simulink model "test2"  (R2020b)
settings: Solver=FixedStepAuto  StartTime=0.0  StopTime=10.0  RelTol=1e-3
model workspace (MAT data in the model file):
  HDLVAXIMasterConfig : hdlverifier.internal.AXIMaster.ConfigParams (value not decoded)
libraries: hdlsllib x38
(part 2 of 2)

== system test2/AesEnc/ram44by32bit/Subsystem ==
  we : Inport  OutDataTypeStr=boolean
  data1 : Inport  Port=2  OutDataTypeStr=uint32
  data2 : Inport  Port=3  OutDataTypeStr=uint32
  Constant : Constant
  Constant1 : Constant  Value=2
  Dual Rate Dual Port RAM : hdlsllib/HDL RAMs/Dual Rate Dual Port RAM  ram_size=2
      settings: SourceProductBaseCode=SL
  temp_state : Outport  OutDataTypeStr=uint32  VectorParamsAs1DForOutWhenUnconnected=off
  temp_state1 : Outport  Port=2  OutDataTypeStr=uint32  VectorParamsAs1DForOutWhenUnconnected=off
  wires:
  Dual Rate Dual Port RAM/1 -> temp_state/1
  data2/1 -> Dual Rate Dual Port RAM/4
  Constant/1 -> Dual Rate Dual Port RAM/2
  data1/1 -> Dual Rate Dual Port RAM/1
  we/1 -> Dual Rate Dual Port RAM/6, Dual Rate Dual Port RAM/3
  Dual Rate Dual Port RAM/2 -> temp_state1/1
  Constant1/1 -> Dual Rate Dual Port RAM/5

== system test2/AesEnc/ram44by32bit/Subsystem1 ==
  we : Inport  OutDataTypeStr=boolean
  data1 : Inport  Port=2  OutDataTypeStr=uint32
  data2 : Inport  Port=3  OutDataTypeStr=uint32
  Constant : Constant
  Constant1 : Constant  Value=2
  Dual Rate Dual Port RAM : hdlsllib/HDL RAMs/Dual Rate Dual Port RAM  ram_size=2
      settings: SourceProductBaseCode=SL
  temp_state : Outport  OutDataTypeStr=uint32  VectorParamsAs1DForOutWhenUnconnected=off
  temp_state1 : Outport  Port=2  OutDataTypeStr=uint32  VectorParamsAs1DForOutWhenUnconnected=off
  wires:
  Dual Rate Dual Port RAM/1 -> temp_state/1
  data2/1 -> Dual Rate Dual Port RAM/4
  Constant/1 -> Dual Rate Dual Port RAM/2
  data1/1 -> Dual Rate Dual Port RAM/1
  we/1 -> Dual Rate Dual Port RAM/6, Dual Rate Dual Port RAM/3
  Dual Rate Dual Port RAM/2 -> temp_state1/1
  Constant1/1 -> Dual Rate Dual Port RAM/5

== system test2/AesEnc/ram44by32bit/Subsystem10 ==
  we : Inport  OutDataTypeStr=boolean
  data1 : Inport  Port=2  OutDataTypeStr=uint32
  data2 : Inport  Port=3  OutDataTypeStr=uint32
  Constant : Constant
  Constant1 : Constant  Value=2
  Dual Rate Dual Port RAM : hdlsllib/HDL RAMs/Dual Rate Dual Port RAM  ram_size=2
      settings: SourceProductBaseCode=SL
  temp_state : Outport  OutDataTypeStr=uint32  VectorParamsAs1DForOutWhenUnconnected=off
  temp_state1 : Outport  Port=2  OutDataTypeStr=uint32  VectorParamsAs1DForOutWhenUnconnected=off
  wires:
  Dual Rate Dual Port RAM/1 -> temp_state/1
  data2/1 -> Dual Rate Dual Port RAM/4
  Constant/1 -> Dual Rate Dual Port RAM/2
  data1/1 -> Dual Rate Dual Port RAM/1
  we/1 -> Dual Rate Dual Port RAM/6, Dual Rate Dual Port RAM/3
  Dual Rate Dual Port RAM/2 -> temp_state1/1
  Constant1/1 -> Dual Rate Dual Port RAM/5

== system test2/AesEnc/ram44by32bit/Subsystem11 ==
  we : Inport  OutDataTypeStr=boolean
  data1 : Inport  Port=2  OutDataTypeStr=uint32
  data2 : Inport  Port=3  OutDataTypeStr=uint32
  Constant : Constant
  Constant1 : Constant  Value=2
  Dual Rate Dual Port RAM : hdlsllib/HDL RAMs/Dual Rate Dual Port RAM  ram_size=2
      settings: SourceProductBaseCode=SL
  temp_state : Outport  OutDataTypeStr=uint32  VectorParamsAs1DForOutWhenUnconnected=off
  temp_state1 : Outport  Port=2  OutDataTypeStr=uint32  VectorParamsAs1DForOutWhenUnconnected=off
  wires:
  Dual Rate Dual Port RAM/1 -> temp_state/1
  data2/1 -> Dual Rate Dual Port RAM/4
  Constant/1 -> Dual Rate Dual Port RAM/2
  data1/1 -> Dual Rate Dual Port RAM/1
  we/1 -> Dual Rate Dual Port RAM/6, Dual Rate Dual Port RAM/3
  Dual Rate Dual Port RAM/2 -> temp_state1/1
  Constant1/1 -> Dual Rate Dual Port RAM/5

== system test2/AesEnc/ram44by32bit/Subsystem12 ==
  we : Inport  OutDataTypeStr=boolean
  data1 : Inport  Port=2  OutDataTypeStr=uint32
  data2 : Inport  Port=3  OutDataTypeStr=uint32
  Constant : Constant
  Constant1 : Constant  Value=2
  Dual Rate Dual Port RAM : hdlsllib/HDL RAMs/Dual Rate Dual Port RAM  ram_size=2
      settings: SourceProductBaseCode=SL
  temp_state : Outport  OutDataTypeStr=uint32  VectorParamsAs1DForOutWhenUnconnected=off
  temp_state1 : Outport  Port=2  OutDataTypeStr=uint32  VectorParamsAs1DForOutWhenUnconnected=off
  wires:
  Dual Rate Dual Port RAM/1 -> temp_state/1
  data2/1 -> Dual Rate Dual Port RAM/4
  Constant/1 -> Dual Rate Dual Port RAM/2
  data1/1 -> Dual Rate Dual Port RAM/1
  we/1 -> Dual Rate Dual Port RAM/6, Dual Rate Dual Port RAM/3
  Dual Rate Dual Port RAM/2 -> temp_state1/1
  Constant1/1 -> Dual Rate Dual Port RAM/5

== system test2/AesEnc/ram44by32bit/Subsystem13 ==
  we : Inport  OutDataTypeStr=boolean
  data1 : Inport  Port=2  OutDataTypeStr=uint32
  data2 : Inport  Port=3  OutDataTypeStr=uint32
  Constant : Constant
  Constant1 : Constant  Value=2
  Dual Rate Dual Port RAM : hdlsllib/HDL RAMs/Dual Rate Dual Port RAM  ram_size=2
      settings: SourceProductBaseCode=SL
  temp_state : Outport  OutDataTypeStr=uint32  VectorParamsAs1DForOutWhenUnconnected=off
  temp_state1 : Outport  Port=2  OutDataTypeStr=uint32  VectorParamsAs1DForOutWhenUnconnected=off
  wires:
  Dual Rate Dual Port RAM/1 -> temp_state/1
  data2/1 -> Dual Rate Dual Port RAM/4
  Constant/1 -> Dual Rate Dual Port RAM/2
  data1/1 -> Dual Rate Dual Port RAM/1
  we/1 -> Dual Rate Dual Port RAM/6, Dual Rate Dual Port RAM/3
  Dual Rate Dual Port RAM/2 -> temp_state1/1
  Constant1/1 -> Dual Rate Dual Port RAM/5

== system test2/AesEnc/ram44by32bit/Subsystem14 ==
  we : Inport  OutDataTypeStr=boolean
  data1 : Inport  Port=2  OutDataTypeStr=uint32
  data2 : Inport  Port=3  OutDataTypeStr=uint32
  Constant : Constant
  Constant1 : Constant  Value=2
  Dual Rate Dual Port RAM : hdlsllib/HDL RAMs/Dual Rate Dual Port RAM  ram_size=2
      settings: SourceProductBaseCode=SL
  temp_state : Outport  OutDataTypeStr=uint32  VectorParamsAs1DForOutWhenUnconnected=off
  temp_state1 : Outport  Port=2  OutDataTypeStr=uint32  VectorParamsAs1DForOutWhenUnconnected=off
  wires:
  Dual Rate Dual Port RAM/1 -> temp_state/1
  data2/1 -> Dual Rate Dual Port RAM/4
  Constant/1 -> Dual Rate Dual Port RAM/2
  data1/1 -> Dual Rate Dual Port RAM/1
  we/1 -> Dual Rate Dual Port RAM/6, Dual Rate Dual Port RAM/3
  Dual Rate Dual Port RAM/2 -> temp_state1/1
  Constant1/1 -> Dual Rate Dual Port RAM/5

== system test2/AesEnc/ram44by32bit/Subsystem15 ==
  we : Inport  OutDataTypeStr=boolean
  data1 : Inport  Port=2  OutDataTypeStr=uint32
  data2 : Inport  Port=3  OutDataTypeStr=uint32
  Constant : Constant
  Constant1 : Constant  Value=2
  Dual Rate Dual Port RAM : hdlsllib/HDL RAMs/Dual Rate Dual Port RAM  ram_size=2
      settings: SourceProductBaseCode=SL
  temp_state : Outport  OutDataTypeStr=uint32  VectorParamsAs1DForOutWhenUnconnected=off
  temp_state1 : Outport  Port=2  OutDataTypeStr=uint32  VectorParamsAs1DForOutWhenUnconnected=off
  wires:
  Dual Rate Dual Port RAM/1 -> temp_state/1
  data2/1 -> Dual Rate Dual Port RAM/4
  Constant/1 -> Dual Rate Dual Port RAM/2
  data1/1 -> Dual Rate Dual Port RAM/1
  we/1 -> Dual Rate Dual Port RAM/6, Dual Rate Dual Port RAM/3
  Dual Rate Dual Port RAM/2 -> temp_state1/1
  Constant1/1 -> Dual Rate Dual Port RAM/5

== system test2/AesEnc/ram44by32bit/Subsystem16 ==
  we : Inport  OutDataTypeStr=boolean
  data1 : Inport  Port=2  OutDataTypeStr=uint32
  data2 : Inport  Port=3  OutDataTypeStr=uint32
  Constant : Constant
  Constant1 : Constant  Value=2
  Dual Rate Dual Port RAM : hdlsllib/HDL RAMs/Dual Rate Dual Port RAM  ram_size=2
      settings: SourceProductBaseCode=SL
  temp_state : Outport  OutDataTypeStr=uint32  VectorParamsAs1DForOutWhenUnconnected=off
  temp_state1 : Outport  Port=2  OutDataTypeStr=uint32  VectorParamsAs1DForOutWhenUnconnected=off
  wires:
  Dual Rate Dual Port RAM/1 -> temp_state/1
  data2/1 -> Dual Rate Dual Port RAM/4
  Constant/1 -> Dual Rate Dual Port RAM/2
  data1/1 -> Dual Rate Dual Port RAM/1
  we/1 -> Dual Rate Dual Port RAM/6, Dual Rate Dual Port RAM/3
  Dual Rate Dual Port RAM/2 -> temp_state1/1
  Constant1/1 -> Dual Rate Dual Port RAM/5

== system test2/AesEnc/ram44by32bit/Subsystem17 ==
  we : Inport  OutDataTypeStr=boolean
  data1 : Inport  Port=2  OutDataTypeStr=uint32
  data2 : Inport  Port=3  OutDataTypeStr=uint32
  Constant : Constant
  Constant1 : Constant  Value=2
  Dual Rate Dual Port RAM : hdlsllib/HDL RAMs/Dual Rate Dual Port RAM  ram_size=2
      settings: SourceProductBaseCode=SL
  temp_state : Outport  OutDataTypeStr=uint32  VectorParamsAs1DForOutWhenUnconnected=off
  temp_state1 : Outport  Port=2  OutDataTypeStr=uint32  VectorParamsAs1DForOutWhenUnconnected=off
  wires:
  Dual Rate Dual Port RAM/1 -> temp_state/1
  data2/1 -> Dual Rate Dual Port RAM/4
  Constant/1 -> Dual Rate Dual Port RAM/2
  data1/1 -> Dual Rate Dual Port RAM/1
  we/1 -> Dual Rate Dual Port RAM/6, Dual Rate Dual Port RAM/3
  Dual Rate Dual Port RAM/2 -> temp_state1/1
  Constant1/1 -> Dual Rate Dual Port RAM/5

== system test2/AesEnc/ram44by32bit/Subsystem18 ==
  we : Inport  OutDataTypeStr=boolean
  data1 : Inport  Port=2  OutDataTypeStr=uint32
  data2 : Inport  Port=3  OutDataTypeStr=uint32
  Constant : Constant
  Constant1 : Constant  Value=2
  Dual Rate Dual Port RAM : hdlsllib/HDL RAMs/Dual Rate Dual Port RAM  ram_size=2
      settings: SourceProductBaseCode=SL
  temp_state : Outport  OutDataTypeStr=uint32  VectorParamsAs1DForOutWhenUnconnected=off
  temp_state1 : Outport  Port=2  OutDataTypeStr=uint32  VectorParamsAs1DForOutWhenUnconnected=off
  wires:
  Dual Rate Dual Port RAM/1 -> temp_state/1
  data2/1 -> Dual Rate Dual Port RAM/4
  Constant/1 -> Dual Rate Dual Port RAM/2
  data1/1 -> Dual Rate Dual Port RAM/1
  we/1 -> Dual Rate Dual Port RAM/6, Dual Rate Dual Port RAM/3
  Dual Rate Dual Port RAM/2 -> temp_state1/1
  Constant1/1 -> Dual Rate Dual Port RAM/5

== system test2/AesEnc/ram44by32bit/Subsystem19 ==
  we : Inport  OutDataTypeStr=boolean
  data1 : Inport  Port=2  OutDataTypeStr=uint32
  data2 : Inport  Port=3  OutDataTypeStr=uint32
  Constant : Constant
  Constant1 : Constant  Value=2
  Dual Rate Dual Port RAM : hdlsllib/HDL RAMs/Dual Rate Dual Port RAM  ram_size=2
      settings: SourceProductBaseCode=SL
  temp_state : Outport  OutDataTypeStr=uint32  VectorParamsAs1DForOutWhenUnconnected=off
  temp_state1 : Outport  Port=2  OutDataTypeStr=uint32  VectorParamsAs1DForOutWhenUnconnected=off
  wires:
  Dual Rate Dual Port RAM/1 -> temp_state/1
  data2/1 -> Dual Rate Dual Port RAM/4
  Constant/1 -> Dual Rate Dual Port RAM/2
  data1/1 -> Dual Rate Dual Port RAM/1
  we/1 -> Dual Rate Dual Port RAM/6, Dual Rate Dual Port RAM/3
  Dual Rate Dual Port RAM/2 -> temp_state1/1
  Constant1/1 -> Dual Rate Dual Port RAM/5

== system test2/AesEnc/ram44by32bit/Subsystem2 ==
  we : Inport  OutDataTypeStr=boolean
  data1 : Inport  Port=2  OutDataTypeStr=uint32
  data2 : Inport  Port=3  OutDataTypeStr=uint32
  Constant : Constant
  Constant1 : Constant  Value=2
  Dual Rate Dual Port RAM : hdlsllib/HDL RAMs/Dual Rate Dual Port RAM  ram_size=2
      settings: SourceProductBaseCode=SL
  temp_state : Outport  OutDataTypeStr=uint32  VectorParamsAs1DForOutWhenUnconnected=off
  temp_state1 : Outport  Port=2  OutDataTypeStr=uint32  VectorParamsAs1DForOutWhenUnconnected=off
  wires:
  Dual Rate Dual Port RAM/1 -> temp_state/1
  data2/1 -> Dual Rate Dual Port RAM/4
  Constant/1 -> Dual Rate Dual Port RAM/2
  data1/1 -> Dual Rate Dual Port RAM/1
  we/1 -> Dual Rate Dual Port RAM/6, Dual Rate Dual Port RAM/3
  Dual Rate Dual Port RAM/2 -> temp_state1/1
  Constant1/1 -> Dual Rate Dual Port RAM/5

== system test2/AesEnc/ram44by32bit/Subsystem20 ==
  we : Inport  OutDataTypeStr=boolean
  data1 : Inport  Port=2  OutDataTypeStr=uint32
  data2 : Inport  Port=3  OutDataTypeStr=uint32
  Constant : Constant
  Constant1 : Constant  Value=2
  Dual Rate Dual Port RAM : hdlsllib/HDL RAMs/Dual Rate Dual Port RAM  ram_size=2
      settings: SourceProductBaseCode=SL
  temp_state : Outport  OutDataTypeStr=uint32  VectorParamsAs1DForOutWhenUnconnected=off
  temp_state1 : Outport  Port=2  OutDataTypeStr=uint32  VectorParamsAs1DForOutWhenUnconnected=off
  wires:
  Dual Rate Dual Port RAM/1 -> temp_state/1
  data2/1 -> Dual Rate Dual Port RAM/4
  Constant/1 -> Dual Rate Dual Port RAM/2
  data1/1 -> Dual Rate Dual Port RAM/1
  we/1 -> Dual Rate Dual Port RAM/6, Dual Rate Dual Port RAM/3
  Dual Rate Dual Port RAM/2 -> temp_state1/1
  Constant1/1 -> Dual Rate Dual Port RAM/5

== system test2/AesEnc/ram44by32bit/Subsystem21 ==
  we : Inport  OutDataTypeStr=boolean
  data1 : Inport  Port=2  OutDataTypeStr=uint32
  data2 : Inport  Port=3  OutDataTypeStr=uint32
  Constant : Constant
  Constant1 : Constant  Value=2
  Dual Rate Dual Port RAM : hdlsllib/HDL RAMs/Dual Rate Dual Port RAM  ram_size=2
      settings: SourceProductBaseCode=SL
  temp_state : Outport  OutDataTypeStr=uint32  VectorParamsAs1DForOutWhenUnconnected=off
  temp_state1 : Outport  Port=2  OutDataTypeStr=uint32  VectorParamsAs1DForOutWhenUnconnected=off
  wires:
  Dual Rate Dual Port RAM/1 -> temp_state/1
  data2/1 -> Dual Rate Dual Port RAM/4
  Constant/1 -> Dual Rate Dual Port RAM/2
  data1/1 -> Dual Rate Dual Port RAM/1
  we/1 -> Dual Rate Dual Port RAM/6, Dual Rate Dual Port RAM/3
  Dual Rate Dual Port RAM/2 -> temp_state1/1
  Constant1/1 -> Dual Rate Dual Port RAM/5

== system test2/AesEnc/ram44by32bit/Subsystem3 ==
  we : Inport  OutDataTypeStr=boolean
  data1 : Inport  Port=2  OutDataTypeStr=uint32
  data2 : Inport  Port=3  OutDataTypeStr=uint32
  Constant : Constant
  Constant1 : Constant  Value=2
  Dual Rate Dual Port RAM : hdlsllib/HDL RAMs/Dual Rate Dual Port RAM  ram_size=2
      settings: SourceProductBaseCode=SL
  temp_state : Outport  OutDataTypeStr=uint32  VectorParamsAs1DForOutWhenUnconnected=off
  temp_state1 : Outport  Port=2  OutDataTypeStr=uint32  VectorParamsAs1DForOutWhenUnconnected=off
  wires:
  Dual Rate Dual Port RAM/1 -> temp_state/1
  data2/1 -> Dual Rate Dual Port RAM/4
  Constant/1 -> Dual Rate Dual Port RAM/2
  data1/1 -> Dual Rate Dual Port RAM/1
  we/1 -> Dual Rate Dual Port RAM/6, Dual Rate Dual Port RAM/3
  Dual Rate Dual Port RAM/2 -> temp_state1/1
  Constant1/1 -> Dual Rate Dual Port RAM/5

== system test2/AesEnc/ram44by32bit/Subsystem4 ==
  we : Inport  OutDataTypeStr=boolean
  data1 : Inport  Port=2  OutDataTypeStr=uint32
  data2 : Inport  Port=3  OutDataTypeStr=uint32
  Constant : Constant
  Constant1 : Constant  Value=2
  Dual Rate Dual Port RAM : hdlsllib/HDL RAMs/Dual Rate Dual Port RAM  ram_size=2
      settings: SourceProductBaseCode=SL
  temp_state : Outport  OutDataTypeStr=uint32  VectorParamsAs1DForOutWhenUnconnected=off
  temp_state1 : Outport  Port=2  OutDataTypeStr=uint32  VectorParamsAs1DForOutWhenUnconnected=off
  wires:
  Dual Rate Dual Port RAM/1 -> temp_state/1
  data2/1 -> Dual Rate Dual Port RAM/4
  Constant/1 -> Dual Rate Dual Port RAM/2
  data1/1 -> Dual Rate Dual Port RAM/1
  we/1 -> Dual Rate Dual Port RAM/6, Dual Rate Dual Port RAM/3
  Dual Rate Dual Port RAM/2 -> temp_state1/1
  Constant1/1 -> Dual Rate Dual Port RAM/5

== system test2/AesEnc/ram44by32bit/Subsystem5 ==
  we : Inport  OutDataTypeStr=boolean
  data1 : Inport  Port=2  OutDataTypeStr=uint32
  data2 : Inport  Port=3  OutDataTypeStr=uint32
  Constant : Constant
  Constant1 : Constant  Value=2
  Dual Rate Dual Port RAM : hdlsllib/HDL RAMs/Dual Rate Dual Port RAM  ram_size=2
      settings: SourceProductBaseCode=SL
  temp_state : Outport  OutDataTypeStr=uint32  VectorParamsAs1DForOutWhenUnconnected=off
  temp_state1 : Outport  Port=2  OutDataTypeStr=uint32  VectorParamsAs1DForOutWhenUnconnected=off
  wires:
  Dual Rate Dual Port RAM/1 -> temp_state/1
  data2/1 -> Dual Rate Dual Port RAM/4
  Constant/1 -> Dual Rate Dual Port RAM/2
  data1/1 -> Dual Rate Dual Port RAM/1
  we/1 -> Dual Rate Dual Port RAM/6, Dual Rate Dual Port RAM/3
  Dual Rate Dual Port RAM/2 -> temp_state1/1
  Constant1/1 -> Dual Rate Dual Port RAM/5

== system test2/AesEnc/ram44by32bit/Subsystem6 ==
  we : Inport  OutDataTypeStr=boolean
  data1 : Inport  Port=2  OutDataTypeStr=uint32
  data2 : Inport  Port=3  OutDataTypeStr=uint32
  Constant : Constant
  Constant1 : Constant  Value=2
  Dual Rate Dual Port RAM : hdlsllib/HDL RAMs/Dual Rate Dual Port RAM  ram_size=2
      settings: SourceProductBaseCode=SL
  temp_state : Outport  OutDataTypeStr=uint32  VectorParamsAs1DForOutWhenUnconnected=off
  temp_state1 : Outport  Port=2  OutDataTypeStr=uint32  VectorParamsAs1DForOutWhenUnconnected=off
  wires:
  Dual Rate Dual Port RAM/1 -> temp_state/1
  data2/1 -> Dual Rate Dual Port RAM/4
  Constant/1 -> Dual Rate Dual Port RAM/2
  data1/1 -> Dual Rate Dual Port RAM/1
  we/1 -> Dual Rate Dual Port RAM/6, Dual Rate Dual Port RAM/3
  Dual Rate Dual Port RAM/2 -> temp_state1/1
  Constant1/1 -> Dual Rate Dual Port RAM/5

== system test2/AesEnc/ram44by32bit/Subsystem7 ==
  we : Inport  OutDataTypeStr=boolean
  data1 : Inport  Port=2  OutDataTypeStr=uint32
  data2 : Inport  Port=3  OutDataTypeStr=uint32
  Constant : Constant
  Constant1 : Constant  Value=2
  Dual Rate Dual Port RAM : hdlsllib/HDL RAMs/Dual Rate Dual Port RAM  ram_size=2
      settings: SourceProductBaseCode=SL
  temp_state : Outport  OutDataTypeStr=uint32  VectorParamsAs1DForOutWhenUnconnected=off
  temp_state1 : Outport  Port=2  OutDataTypeStr=uint32  VectorParamsAs1DForOutWhenUnconnected=off
  wires:
  Dual Rate Dual Port RAM/1 -> temp_state/1
  data2/1 -> Dual Rate Dual Port RAM/4
  Constant/1 -> Dual Rate Dual Port RAM/2
  data1/1 -> Dual Rate Dual Port RAM/1
  we/1 -> Dual Rate Dual Port RAM/6, Dual Rate Dual Port RAM/3
  Dual Rate Dual Port RAM/2 -> temp_state1/1
  Constant1/1 -> Dual Rate Dual Port RAM/5

== system test2/AesEnc/ram44by32bit/Subsystem8 ==
  we : Inport  OutDataTypeStr=boolean
  data1 : Inport  Port=2  OutDataTypeStr=uint32
  data2 : Inport  Port=3  OutDataTypeStr=uint32
  Constant : Constant
  Constant1 : Constant  Value=2
  Dual Rate Dual Port RAM : hdlsllib/HDL RAMs/Dual Rate Dual Port RAM  ram_size=2
      settings: SourceProductBaseCode=SL
  temp_state : Outport  OutDataTypeStr=uint32  VectorParamsAs1DForOutWhenUnconnected=off
  temp_state1 : Outport  Port=2  OutDataTypeStr=uint32  VectorParamsAs1DForOutWhenUnconnected=off
  wires:
  Dual Rate Dual Port RAM/1 -> temp_state/1
  data2/1 -> Dual Rate Dual Port RAM/4
  Constant/1 -> Dual Rate Dual Port RAM/2
  data1/1 -> Dual Rate Dual Port RAM/1
  we/1 -> Dual Rate Dual Port RAM/6, Dual Rate Dual Port RAM/3
  Dual Rate Dual Port RAM/2 -> temp_state1/1
  Constant1/1 -> Dual Rate Dual Port RAM/5

== system test2/AesEnc/ram44by32bit/Subsystem9 ==
  we : Inport  OutDataTypeStr=boolean
  data1 : Inport  Port=2  OutDataTypeStr=uint32
  data2 : Inport  Port=3  OutDataTypeStr=uint32
  Constant : Constant
  Constant1 : Constant  Value=2
  Dual Rate Dual Port RAM : hdlsllib/HDL RAMs/Dual Rate Dual Port RAM  ram_size=2
      settings: SourceProductBaseCode=SL
  temp_state : Outport  OutDataTypeStr=uint32  VectorParamsAs1DForOutWhenUnconnected=off
  temp_state1 : Outport  Port=2  OutDataTypeStr=uint32  VectorParamsAs1DForOutWhenUnconnected=off
  wires:
  Dual Rate Dual Port RAM/1 -> temp_state/1
  data2/1 -> Dual Rate Dual Port RAM/4
  Constant/1 -> Dual Rate Dual Port RAM/2
  data1/1 -> Dual Rate Dual Port RAM/1
  we/1 -> Dual Rate Dual Port RAM/6, Dual Rate Dual Port RAM/3
  Dual Rate Dual Port RAM/2 -> temp_state1/1
  Constant1/1 -> Dual Rate Dual Port RAM/5

== matlab function test2/AesEnc/MATLAB Function ==
  data: message_type input; load_key output; load_state output; expand_key output; run_enc output; enc_complete output; busy input; loadkey_complete input; loadstate_complete input; expandkey_complete input; runenc_complete input; enccomplete_complete input; disable output
function [load_key, load_state, expand_key, run_enc, enc_complete, disable] = AESEnc_state_machine(message_type, busy, loadkey_complete, loadstate_complete, expandkey_complete, runenc_complete, enccomplete_complete)
%     inputs
%     in_stream 128, message_type 8, enable 1
%     outputs
%     out_stream 128, complete 1
        
%     state 0 waiting for input
%     state 1 is enable turned on
%     state 2 is key loaded
%     state 3 is state loaded
%     state 4 is run the key expansion
%     state 5 is run the encryption
%     state 6 is encryption complete
    
    if (busy == boolean(1) && message_type == uint8('1'))
        load_key = boolean(1);
        load_state = boolean(0);
        expand_key = boolean(0);
        run_enc = boolean(0);
        enc_complete = boolean(0);
        disable = boolean(0);
    end
    
    if (loadkey_complete == boolean(1) && message_type == uint8('2'))
%         input is a state
        load_key = boolean(0);
        load_state = boolean(1);
        expand_key = boolean(0);
        run_enc = boolean(0);
        enc_complete = boolean(0);
        disable = boolean(0);
    end
    
    if (loadstate_complete == boolean(1))
        load_key = boolean(0);
        load_state = boolean(0);
        expand_key = boolean(1);
        run_enc = boolean(0);
        enc_complete = boolean(0);
        disable = boolean(0);
    end
    
    if (expandkey_complete == boolean(1))
        load_key = boolean(0);
        load_state = boolean(0);
        expand_key = boolean(0);
        run_enc = boolean(1);
        enc_complete = boolean(0);
        disable = boolean(0);
    end
    
    if (runenc_complete == boolean(1))
        load_key = boolean(0);
        load_state = boolean(0);
        expand_key = boolean(0);
        run_enc = boolean(0);
        enc_complete = boolean(1);
        disable = boolean(0);
    end
    
    if (enccomplete_complete == boolean(1))
        load_key = boolean(0);
        load_state = boolean(0);
        expand_key = boolean(0);
        run_enc = boolean(0);
        enc_complete = boolean(0);
        disable = boolean(1);
    end
end

== matlab function test2/AesEnc/KeyExpansion ==
  data: complete output; enable input; key1 input; w1 output; key2 input; key3 input; key4 input; key5 input; key6 input; key7 input; key8 input; key9 input; key10 input; key11 input; key12 input; key13 input; key14 input; key15 input; key16 input; w2 output; w3 output; w4 output; w5 output; w6 output; w7 output; w8 output; w9 output; w10 output; w11 output; w12 output; w13 output; w14 output; w15 output; w16 output; w17 output; w18 output; w19 output; w20 output; w21 output; w22 output; w23 output; w24 output; w25 output; w26 output; w27 output; w28 output; w29 output; w30 output; w31 output; w32 output; w33 output; w34 output; w35 output; w36 output; w37 output; w38 output; w39 output; w40 output; w41 output; w42 output; w43 output; w44 output
function [complete, w1, w2, w3, w4, w5, w6, w7, w8, w9, w10, w11, w12, w13, w14, w15, w16, w17, w18, w19, w20, w21, w22, w23, w24, w25, w26, w27, w28, w29, w30, w31, w32, w33, w34, w35, w36, w37, w38, w39, w40, w41, w42, w43, w44] = KeyExpansion(enable, key1, key2, key3, key4, key5, key6, key7, key8, key9, key10, key11, key12, key13, key14, key15, key16)

if (enable == boolean(1))
%     round constant do not delete
    Rcon = uint32([0x8d000000 0x01000000 0x02000000 0x04000000 0x08000000 0x10000000 0x20000000 0x40000000 0x80000000 0x1b000000 0x36000000 ]);
    
    w = uint32(zeros(1,44));
% 	temp = uint32(0);
% 	i = uint8(1);

    % first loop worked out:

    % iteration 1:
    w(1) = w(1) + uint32(key1);
    w(1) = bitsll(w(1), 8);
    w(1) = w(1) + uint32(key2);
    w(1) = bitsll(w(1), 8);
    w(1) = w(1) + uint32(key3);
    w(1) = bitsll(w(1), 8);
    w(1) = w(1) + uint32(key4);

    % iteration 2:
    w(2) = w(2) + uint32(key5);
    w(2) = bitsll(w(2), 8);
    w(2) = w(2) + uint32(key6);
    w(2) = bitsll(w(2), 8);
    w(2) = w(2) + uint32(key7);
    w(2) = bitsll(w(2), 8);
    w(2) = w(2) + uint32(key8);

    % iteration 3:
    w(3) = w(3) + uint32(key9);
    w(3) = bitsll(w(3), 8);
    w(3) = w(3) + uint32(key10);
    w(3) = bitsll(w(3), 8);
    w(3) = w(3) + uint32(key11);
    w(3) = bitsll(w(3), 8);
    w(3) = w(3) + uint32(key12);

    % iteration 4:
    w(4) = w(4) + uint32(key13);
    w(4) = bitsll(w(4), 8);
    w(4) = w(4) + uint32(key14);
    w(4) = bitsll(w(4), 8);
    w(4) = w(4) + uint32(key15);
    w(4) = bitsll(w(4), 8);
    w(4) = w(4) + uint32(key16);

%     %the rest of the blocks
%     for i = 4:43
% 		temp = uint32(w(i));
%         if (mod(i, 4) == 0) % this has been changed 
% 			temp = uint32(RotWord(temp));
% 			temp = uint32(SubWord(temp));
% 			temp = uint32(bitxor(temp, Rcon(floor((i+1) / 4 )+1))); % might need to be i + 1
%         end
% 		w(i+1) = bitxor(w(i - 3), temp);
%     end
	
    w1 = w(1);
    w2 = w(2);
    w3 = w(3);
    w4 = w(4); 
    
    w(5) = w(4);
    w(5) = uint32(RotWord(w(5)));
    w(5) = uint32(SubWord(w(5)));
    w(5) = uint32(bitxor(w(5), Rcon(2)));
    w(5) = bitxor(w(1), w(5));    
    w5 = w(5);
    
    w(6) = bitxor(w(5), w(2));
    w6 = w(6);
    w(7) = bitxor(w(6), w(3));
    w7 = w(7);
    w(8) = bitxor(w(7), w(4));
    w8 = w(8);

    w(9) = w(8);
    w(9) = uint32(RotWord(w(9)));
    w(9) = uint32(SubWord(w(9)));
    w(9) = uint32(bitxor(w(9), Rcon(3))); 
    w(9) = bitxor(w(5), w(9));
    w9 = w(9);
     
    w(10) = bitxor(w(9), w(6));
    w10 = w(10);
    w(11) = bitxor(w(10), w(7));
    w11 = w(11);
    w(12) = bitxor(w(11), w(8));
    w12 = w(12);
    
    w(13) = w(12);
    w(13) = uint32(RotWord(w(13)));
    w(13) = uint32(SubWord(w(13)));
    w(13) = uint32(bitxor(w(13), Rcon(4))); 
    w(13) = bitxor(w(9), w(13));
    w13 = w(13);

    w(14) = bitxor(w(13), w(10));
    w14 = w(14);
    w(15) = bitxor(w(14), w(11));
    w15 = w(15);
    w(16) = bitxor(w(15), w(12));
    w16 = w(16);
    
    w(17) = w(16);
    w(17) = uint32(RotWord(w(17)));
    w(17) = uint32(SubWord(w(17)));
    w(17) = uint32(bitxor(w(17), Rcon(5))); 
    w(17) = bitxor(w(13), w(17));
    w17 = w(17);
    
    w(18) = bitxor(w(17), w(14));
    w18 = w(18);
    w(19) = bitxor(w(18), w(15));
    w19 = w(19);
    w(20) = bitxor(w(19), w(16));
    w20 = w(20);
    
    w(21) = w(20);
    w(21) = uint32(RotWord(w(21)));
    w(21) = uint32(SubWord(w(21)));
    w(21) = uint32(bitxor(w(21), Rcon(6))); 
    w(21) = bitxor(w(17), w(21));
    w21 = w(21);
    
    w(22) = bitxor(w(21), w(18));
    w22 = w(22);
    w(23) = bitxor(w(22), w(19));
    w23 = w(23);
    w(24) = bitxor(w(23), w(20));
    w24 = w(24);
    
    w(25) = w(24);
    w(25) = uint32(RotWord(w(25)));
    w(25) = uint32(SubWord(w(25)));
    w(25) = uint32(bitxor(w(25), Rcon(7))); 
    w(25) = bitxor(w(21), w(25));
    w25 = w(25);
    
    w(26) = bitxor(w(25), w(22));
    w26 = w(26);
    w(27) = bitxor(w(26), w(23));
    w27 = w(27);
    w(28) = bitxor(w(27), w(24));
    w28 = w(28);
    
    w(29) = w(28);
    w(29) = uint32(RotWord(w(29)));
    w(29) = uint32(SubWord(w(29)));
    w(29) = uint32(bitxor(w(29), Rcon(8))); 
    w(29) = bitxor(w(25), w(29));
    w29 = w(29);
    
    w(30) = bitxor(w(29), w(26));
    w30 = w(30);
    w(31) = bitxor(w(30), w(27));
    w31 = w(31);
    w(32) = bitxor(w(31), w(28));
    w32 = w(32);
    
    w(33) = w(32);
    w(33) = uint32(RotWord(w(33)));
    w(33) = uint32(SubWord(w(33)));
    w(33) = uint32(bitxor(w(33), Rcon(9))); 
    w(33) = bitxor(w(29), w(33));
    w33 = w(33);
   
    w(34) = bitxor(w(33), w(30));
    w34 = w(34);
    w(35) = bitxor(w(34), w(31));
    w35 = w(35);
    w(36) = bitxor(w(35), w(32));
    w36 = w(36);
    
    w(37) = w(36);
    w(37) = uint32(RotWord(w(37)));
    w(37) = uint32(SubWord(w(37)));
    w(37) = uint32(bitxor(w(37), Rcon(10))); 
    w(37) = bitxor(w(33), w(37));
    w37 = w(37);
    
    w(38) = bitxor(w(37), w(34));
    w38 = w(38);
    w(39) = bitxor(w(38), w(35));
    w39 = w(39);
    w(40) = bitxor(w(39), w(36));
    w40 = w(40);
    
    w(41) = w(40);
    w(41) = uint32(RotWord(w(41)));
    w(41) = uint32(SubWord(w(41)));
    w(41) = uint32(bitxor(w(41), Rcon(11))); 
    w(41) = bitxor(w(37), w(41));
    w41 = w(41);
    
    w(42) = bitxor(w(41), w(38));
    w42 = w(42);
    w(43) = bitxor(w(42), w(39));
    w43 = w(43);
    w(44) = bitxor(w(43), w(40));
    w44 = w(44);
    
    complete = boolean(1);
else
    complete = boolean(0);
end
end

== matlab function test2/AesEnc/KeyEschedule ==
  data: key1 output; key2 output; key3 output; key4 output; key5 output; key6 output; key7 output; key8 output; key9 output; key10 output; key11 output; key12 output; key13 output; key14 output; key15 output; key16 output; w1 input; w2 input; w3 input; w4 input; w5 input; w6 input; w7 input; w8 input; w9 input; w10 input; w11 input; w12 input; w13 input; w14 input; w15 input; w16 input; w17 input; w18 input; w19 input; w20 input; w21 input; w22 input; w23 input; w24 input; w25 input; w26 input; w27 input; w28 input; w29 input; w30 input; w31 input; w32 input; w33 input; w34 input; w35 input; w36 input; w37 input; w38 input; w39 input; w40 input; w41 input; w42 input; w43 input; w44 input; XTime_out output; start input; XTime input; busy output
function [key1, key2, key3, key4, key5, key6, key7, key8, key9, key10, key11, key12, key13, key14, key15, key16, XTime_out, busy] = KeyEschedule(w1, w2, w3, w4, w5, w6, w7, w8, w9, w10, w11, w12, w13, w14, w15, w16, w17, w18, w19, w20, w21, w22, w23, w24, w25, w26, w27, w28, w29, w30, w31, w32, w33, w34, w35, w36, w37, w38, w39, w40, w41, w42, w43, w44, start, XTime)
    % keys are 8 bits each
    % ws are 32 bits each

    if (start == boolean(1) && XTime == uint8(0))
        key1 = bitsrl(w1, 24);
        key2 = bitsrl(bitsll(w1, 8), 24);
        key3 = bitsrl(bitsll(w1, 16), 24);
        key4 = bitsrl(bitsll(w1, 24), 24);        
        key5 = bitsrl(w2, 24);
        key6 = bitsrl(bitsll(w2, 8), 24);
        key7 = bitsrl(bitsll(w2, 16), 24);
        key8 = bitsrl(bitsll(w2, 24), 24);
        key9 = bitsrl(w3, 24);
        key10 = bitsrl(bitsll(w3, 8), 24);
        key11 = bitsrl(bitsll(w3, 16), 24);
        key12 = bitsrl(bitsll(w3, 24), 24);
        key13 = bitsrl(w4, 24);
        key14 = bitsrl(bitsll(w4, 8), 24);
        key15 = bitsrl(bitsll(w4, 16), 24);
        key16 = bitsrl(bitsll(w4, 24), 24);
        XTime_out = uint8(0);
        busy = boolean(1);
    end
    
    if (XTime == uint8(1))
        key1 = bitsrl(w5, 24);
        key2 = bitsrl(bitsll(w5, 8), 24);
        key3 = bitsrl(bitsll(w5, 16), 24);
        key4 = bitsrl(bitsll(w5, 24), 24);        
        key5 = bitsrl(w6, 24);
        key6 = bitsrl(bitsll(w6, 8), 24);
        key7 = bitsrl(bitsll(w6, 16), 24);
        key8 = bitsrl(bitsll(w6, 24), 24);
        key9 = bitsrl(w7, 24);
        key10 = bitsrl(bitsll(w7, 8), 24);
        key11 = bitsrl(bitsll(w7, 16), 24);
        key12 = bitsrl(bitsll(w7, 24), 24);
        key13 = bitsrl(w8, 24);
        key14 = bitsrl(bitsll(w8, 8), 24);
        key15 = bitsrl(bitsll(w8, 16), 24);
        key16 = bitsrl(bitsll(w8, 24), 24);
    elseif (XTime == uint8(2))
        key1 = bitsrl(w9, 24);
        key2 = bitsrl(bitsll(w9, 8), 24);
        key3 = bitsrl(bitsll(w9, 16), 24);
        key4 = bitsrl(bitsll(w9, 24), 24);        
        key5 = bitsrl(w10, 24);
        key6 = bitsrl(bitsll(w10, 8), 24);
        key7 = bitsrl(bitsll(w10, 16), 24);
        key8 = bitsrl(bitsll(w10, 24), 24);
        key9 = bitsrl(w11, 24);
        key10 = bitsrl(bitsll(w11, 8), 24);
        key11 = bitsrl(bitsll(w11, 16), 24);
        key12 = bitsrl(bitsll(w11, 24), 24);
        key13 = bitsrl(w12, 24);
        key14 = bitsrl(bitsll(w12, 8), 24);
        key15 = bitsrl(bitsll(w12, 16), 24);
        key16 = bitsrl(bitsll(w12, 24), 24);
    elseif (XTime == uint8(3))
        key1 = bitsrl(w13, 24);
        key2 = bitsrl(bitsll(w13, 8), 24);
        key3 = bitsrl(bitsll(w13, 16), 24);
        key4 = bitsrl(bitsll(w13, 24), 24);        
        key5 = bitsrl(w14, 24);
        key6 = bitsrl(bitsll(w14, 8), 24);
        key7 = bitsrl(bitsll(w14, 16), 24);
        key8 = bitsrl(bitsll(w14, 24), 24);
        key9 = bitsrl(w15, 24);
        key10 = bitsrl(bitsll(w15, 8), 24);
        key11 = bitsrl(bitsll(w15, 16), 24);
        key12 = bitsrl(bitsll(w15, 24), 24);
        key13 = bitsrl(w16, 24);
        key14 = bitsrl(bitsll(w16, 8), 24);
        key15 = bitsrl(bitsll(w16, 16), 24);
        key16 = bitsrl(bitsll(w16, 24), 24);
    elseif (XTime == uint8(4))
        key1 = bitsrl(w17, 24);
        key2 = bitsrl(bitsll(w17, 8), 24);
        key3 = bitsrl(bitsll(w17, 16), 24);
        key4 = bitsrl(bitsll(w17, 24), 24);        
        key5 = bitsrl(w18, 24);
        key6 = bitsrl(bitsll(w18, 8), 24);
        key7 = bitsrl(bitsll(w18, 16), 24);
        key8 = bitsrl(bitsll(w18, 24), 24);
        key9 = bitsrl(w19, 24);
        key10 = bitsrl(bitsll(w19, 8), 24);
        key11 = bitsrl(bitsll(w19, 16), 24);
        key12 = bitsrl(bitsll(w19, 24), 24);
        key13 = bitsrl(w20, 24);
        key14 = bitsrl(bitsll(w20, 8), 24);
        key15 = bitsrl(bitsll(w20, 16), 24);
        key16 = bitsrl(bitsll(w20, 24), 24);
    elseif (XTime == uint8(5))
        key1 = bitsrl(w21, 24);
        key2 = bitsrl(bitsll(w21, 8), 24);
        key3 = bitsrl(bitsll(w21, 16), 24);
        key4 = bitsrl(bitsll(w21, 24), 24);        
        key5 = bitsrl(w22, 24);
        key6 = bitsrl(bitsll(w22, 8), 24);
        key7 = bitsrl(bitsll(w22, 16), 24);
        key8 = bitsrl(bitsll(w22, 24), 24);
        key9 = bitsrl(w23, 24);
        key10 = bitsrl(bitsll(w23, 8), 24);
        key11 = bitsrl(bitsll(w23, 16), 24);
        key12 = bitsrl(bitsll(w23, 24), 24);
        key13 = bitsrl(w24, 24);
        key14 = bitsrl(bitsll(w24, 8), 24);
        key15 = bitsrl(bitsll(w24, 16), 24);
        key16 = bitsrl(bitsll(w24, 24), 24);
    elseif (XTime == uint8(6))
        key1 = bitsrl(w25, 24);
        key2 = bitsrl(bitsll(w25, 8), 24);
        key3 = bitsrl(bitsll(w25, 16), 24);
        key4 = bitsrl(bitsll(w25, 24), 24);        
        key5 = bitsrl(w26, 24);
        key6 = bitsrl(bitsll(w26, 8), 24);
        key7 = bitsrl(bitsll(w26, 16), 24);
        key8 = bitsrl(bitsll(w26, 24), 24);
        key9 = bitsrl(w27, 24);
        key10 = bitsrl(bitsll(w27, 8), 24);
        key11 = bitsrl(bitsll(w27, 16), 24);
        key12 = bitsrl(bitsll(w27, 24), 24);
        key13 = bitsrl(w28, 24);
        key14 = bitsrl(bitsll(w28, 8), 24);
        key15 = bitsrl(bitsll(w28, 16), 24);
        key16 = bitsrl(bitsll(w28, 24), 24);
    elseif (XTime == uint8(7))
        key1 = bitsrl(w29, 24);
        key2 = bitsrl(bitsll(w29, 8), 24);
        key3 = bitsrl(bitsll(w29, 16), 24);
        key4 = bitsrl(bitsll(w29, 24), 24);        
        key5 = bitsrl(w30, 24);
        key6 = bitsrl(bitsll(w30, 8), 24);
        key7 = bitsrl(bitsll(w30, 16), 24);
        key8 = bitsrl(bitsll(w30, 24), 24);
        key9 = bitsrl(w31, 24);
        key10 = bitsrl(bitsll(w31, 8), 24);
        key11 = bitsrl(bitsll(w31, 16), 24);
        key12 = bitsrl(bitsll(w31, 24), 24);
        key13 = bitsrl(w32, 24);
        key14 = bitsrl(bitsll(w32, 8), 24);
        key15 = bitsrl(bitsll(w32, 16), 24);
        key16 = bitsrl(bitsll(w32, 24), 24);
    elseif (XTime == uint8(8))
        key1 = bitsrl(w33, 24);
        key2 = bitsrl(bitsll(w33, 8), 24);
        key3 = bitsrl(bitsll(w33, 16), 24);
        key4 = bitsrl(bitsll(w33, 24), 24);        
        key5 = bitsrl(w34, 24);
        key6 = bitsrl(bitsll(w34, 8), 24);
        key7 = bitsrl(bitsll(w34, 16), 24);
        key8 = bitsrl(bitsll(w34, 24), 24);
        key9 = bitsrl(w35, 24);
        key10 = bitsrl(bitsll(w35, 8), 24);
        key11 = bitsrl(bitsll(w35, 16), 24);
        key12 = bitsrl(bitsll(w35, 24), 24);
        key13 = bitsrl(w36, 24);
        key14 = bitsrl(bitsll(w36, 8), 24);
        key15 = bitsrl(bitsll(w36, 16), 24);
        key16 = bitsrl(bitsll(w36, 24), 24);
    elseif (XTime == uint8(9))
        key1 = bitsrl(w37, 24);
        key2 = bitsrl(bitsll(w37, 8), 24);
        key3 = bitsrl(bitsll(w37, 16), 24);
        key4 = bitsrl(bitsll(w37, 24), 24);        
        key5 = bitsrl(w38, 24);
        key6 = bitsrl(bitsll(w38, 8), 24);
        key7 = bitsrl(bitsll(w38, 16), 24);
        key8 = bitsrl(bitsll(w38, 24), 24);
        key9 = bitsrl(w39, 24);
        key10 = bitsrl(bitsll(w39, 8), 24);
        key11 = bitsrl(bitsll(w39, 16), 24);
        key12 = bitsrl(bitsll(w39, 24), 24);
        key13 = bitsrl(w40, 24);
        key14 = bitsrl(bitsll(w40, 8), 24);
        key15 = bitsrl(bitsll(w40, 16), 24);
        key16 = bitsrl(bitsll(w40, 24), 24);
    elseif (XTime == uint8(10))
        key1 = bitsrl(w41, 24);
        key2 = bitsrl(bitsll(w41, 8), 24);
        key3 = bitsrl(bitsll(w41, 16), 24);
        key4 = bitsrl(bitsll(w41, 24), 24);        
        key5 = bitsrl(w42, 24);
        key6 = bitsrl(bitsll(w42, 8), 24);
        key7 = bitsrl(bitsll(w42, 16), 24);
        key8 = bitsrl(bitsll(w42, 24), 24);
        key9 = bitsrl(w43, 24);
        key10 = bitsrl(bitsll(w43, 8), 24);
        key11 = bitsrl(bitsll(w43, 16), 24);
        key12 = bitsrl(bitsll(w43, 24), 24);
        key13 = bitsrl(w44, 24);
        key14 = bitsrl(bitsll(w44, 8), 24);
        key15 = bitsrl(bitsll(w44, 16), 24);
        key16 = bitsrl(bitsll(w44, 24), 24);
    else
        busy = boolean(0);
    end
end

== matlab function test2/AesEnc/MATLAB Function1 ==
  data: enable input; busy output; disable input
function busy  = enc_running(enable, disable)
    busy = boolean(0);
    
    if (enable == true)
        busy = boolean(1);
    end
    
    if (disable == true)
        busy = boolean(0);
    end
    
end

== matlab function test2/AesEnc/RunEnc ==
  data: state_out1 output; state_out2 output; state_out3 output; state_out4 output; state_out5 output; state_out6 output; state_out7 output; state_out8 output; state_out9 output; state_out10 output; state_out11 output; state_out12 output; state_out13 output; state_out14 output; state_out15 output; state_out16 output; key1 input; key2 input; key3 input; key4 input; key5 input; key6 input; key7 input; key8 input; key9 input; key10 input; key11 input; key12 input; key13 input; key14 input; key15 input; key16 input; XTime_out output; state1 input; state2 input; state3 input; state4 input; state5 input; state6 input; state7 input; state8 input; state9 input; state10 input; state11 input; state12 input; state13 input; state14 input; state15 input; state16 input; XTime input; enable input
function [state_out1, state_out2, state_out3, state_out4, state_out5, state_out6, state_out7, state_out8, state_out9, state_out10, state_out11, state_out12, state_out13, state_out14, state_out15, state_out16, XTime_out] = RunEnc(key1, key2, key3, key4, key5, key6, key7, key8, key9, key10, key11, key12, key13, key14, key15, key16, state1, state2, state3, state4, state5, state6, state7, state8, state9, state10, state11, state12, state13, state14, state15, state16, XTime, enable)
    % keys are 8 bits each
    % ws are 32 bits each
    
    state = uint8([state1, state2, state3, state4, state5, state6, state7, state8, state9, state10, state11, state12, state13, state14, state15, state16]);
    key = uint8([key1, key2, key3, key4, key5, key6, key7, key8, key9, key10, key11, key12, key13, key14, key15, key16]);
    if (enable == boolean(1))    
    if (XTime == uint8(0))
        state = addKey(state, key);
        XTime_out = uint8(1);
    elseif (XTime == uint8(1))
        %subbytes
        state = SubBytes(state);
        %shift rows
        state = ShiftRows(state);
        %mix columns
        state = MixColumns(state);
        %XOR with key
        state = addKey(state, key);
        XTime_out = uint8(2);
    elseif (XTime == uint8(2))
        %subbytes
        state = SubBytes(state);
        %shift rows
        state = ShiftRows(state);
        %mix columns
        state = MixColumns(state);
        %XOR with key
        state = addKey(state, key);
        XTime_out = uint8(3);
    elseif (XTime == uint8(3))
        %subbytes
        state = SubBytes(state);
        %shift rows
        state = ShiftRows(state);
        %mix columns
        state = MixColumns(state);
        %XOR with key
        state = addKey(state, key);
        XTime_out = uint8(4);
    elseif (XTime == uint8(4))
        %subbytes
        state = SubBytes(state);
        %shift rows
        state = ShiftRows(state);
        %mix columns
        state = MixColumns(state);
        %XOR with key
        state = addKey(state, key);
        XTime_out = uint8(5);
    elseif (XTime == uint8(5))
        %subbytes
        state = SubBytes(state);
        %shift rows
        state = ShiftRows(state);
        %mix columns
        state = MixColumns(state);
        %XOR with key
        state = addKey(state, key);
        XTime_out = uint8(6);
    elseif (XTime == uint8(6))
        %subbytes
        state = SubBytes(state);
        %shift rows
        state = ShiftRows(state);
        %mix columns
        state = MixColumns(state);
        %XOR with key
        state = addKey(state, key);
        XTime_out = uint8(7);
    elseif (XTime == uint8(7))
        %subbytes
        state = SubBytes(state);
        %shift rows
        state = ShiftRows(state);
        %mix columns
        state = MixColumns(state);
        %XOR with key
        state = addKey(state, key);
        XTime_out = uint8(8);
    elseif (XTime == uint8(8))
        %subbytes
        state = SubBytes(state);
        %shift rows
        state = ShiftRows(state);
        %mix columns
        state = MixColumns(state);
        %XOR with key
        state = addKey(state, key);
        XTime_out = uint8(9);
    elseif (XTime == uint8(9))
        %subbytes
        state = SubBytes(state);
        %shift rows
        state = ShiftRows(state);
        %mix columns
        state = MixColumns(state);
        %XOR with key
        state = addKey(state, key);
        XTime_out = uint8(10);
    elseif (XTime == uint8(10))
        %subbytes
        state = SubBytes(state);
        %shift rows
        state = ShiftRows(state);
        %mix columns
        %state = MixColumns(state);
        %XOR with key
        state = addKey(state, key);
        XTime_out = uint8(11);
    end
    
    state_out1 = state(1);
    state_out2 = state(2);
    state_out3 = state(3);
    state_out4 = state(4);
    state_out5 = state(5);
    state_out6 = state(6);
    state_out7 = state(7);
    state_out8 = state(8);
    state_out9 = state(9);
    state_out10 = state(10);
    state_out11 = state(11);
    state_out12 = state(12);
    state_out13 = state(13);
    state_out14 = state(14);
    state_out15 = state(15);
    state_out16 = state(16);
    end
end

== matlab function test2/RunEnc ==
  data: ret_word output; word input
function ret_word  = RotWord(word)
	%rotate word for KeyExpansion
	%B1 -> B4
	%B2 -> B1
	%B3 -> B2
	%B4 -> B3
%       // 4  3  2  1
%       // 3c 4f cf 09
%       // cf 4f 3c 09
    words = zeros(1, 4, 'uint32');
    words(4) = bitsrl(bitand(word, 0xFF000000), 24);
    words(3) = bitsrl(bitsll(bitand(word, 0x00FF0000), 8), 24);
    words(2) = bitsrl(bitsll(bitand(word, 0x0000FF00), 16), 24);
    words(1) = bitsrl(bitsll(bitand(word, 0x000000FF), 24), 24);
	
    ret_word = uint32(0);
    
	ret_word = ret_word + words(3);
	ret_word = bitsll(ret_word, 8);
	ret_word = ret_word + words(2);
	ret_word = bitsll(ret_word, 8);
	ret_word = ret_word + words(1);
	ret_word = bitsll(ret_word, 8);
	ret_word = ret_word + words(4);
end
